simulink model "joystick_pr"  (R2021a)
settings: Solver=VariableStepAuto  StartTime=0.0  StopTime=Inf  RelTol=1e-3
libraries: vrlib x1, aerolibanimutils x1
settings Model: Creator=Samsung  LastModifiedBy=Samsung

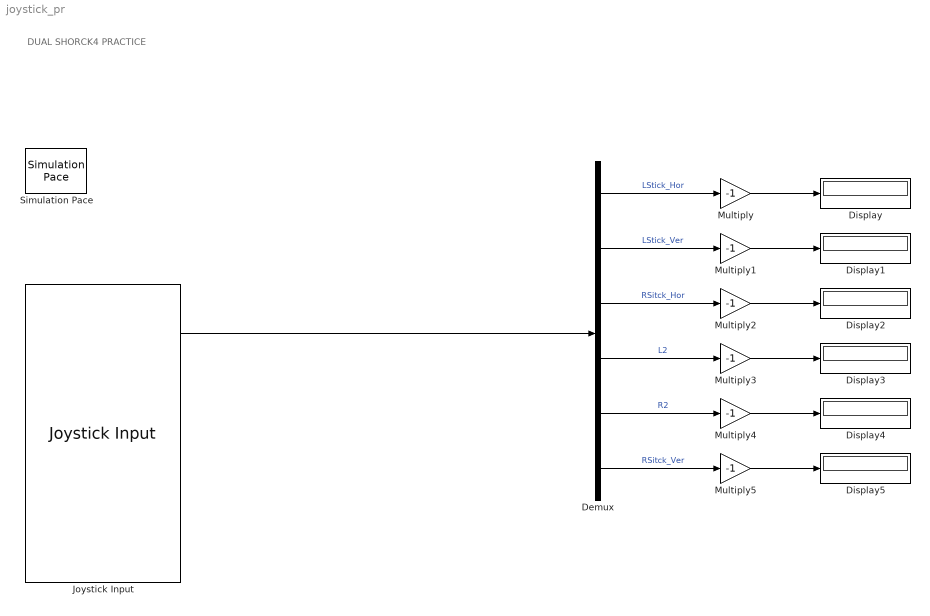
== system joystick_pr ==
  note: DUAL SHORCK4 PRACTICE
  Demux : Demux  Outputs=6
  Display{,1..5} (6 alike) : Display
  Joystick Input : vrlib/Joystick Input  joyid=1  adjustports=on  forcefeed=off
  Multiply{,1..5} (6 alike) : Gain  Gain=-1
  Simulation Pace : aerolibanimutils/Simulation Pace  SimulationPace=1  SleepMode=Auto  OutputPaceError=off  SampleTime=1/30
  wires:
  Joystick Input/1 -> Demux/1
  Demux/1 -> Multiply/1  "LStick_Hor"
  Demux/2 -> Multiply1/1  "LStick_Ver"
  Demux/3 -> Multiply2/1  "RSitck_Hor"
  Demux/5 -> Multiply4/1  "R2"
  Demux/6 -> Multiply5/1  "RSitck_Ver"
  Demux/4 -> Multiply3/1  "L2"
  Multiply/1 -> Display/1
  Multiply1/1 -> Display1/1
  Multiply2/1 -> Display2/1
  Multiply3/1 -> Display3/1
  Multiply4/1 -> Display4/1
  Multiply5/1 -> Display5/1
